simulink model "Threephase_diode_bridge_rectifier"  (R2022b)
settings: Solver=VariableStepAuto  StartTime=0.0  StopTime=10.0  RelTol=1e-3
libraries: spsDiodeLib x6, spsACVoltageSourceLib x3, spsMultimeterLib x3, spsSeriesRLCBranchLib x1, sps_lib x1
settings Model: Creator=vs632  LastModifiedBy=vs632

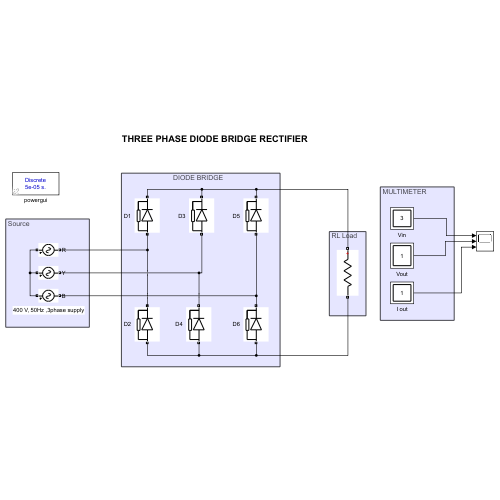
[thumbnail: Simulink's stored preview of the top-level diagram]
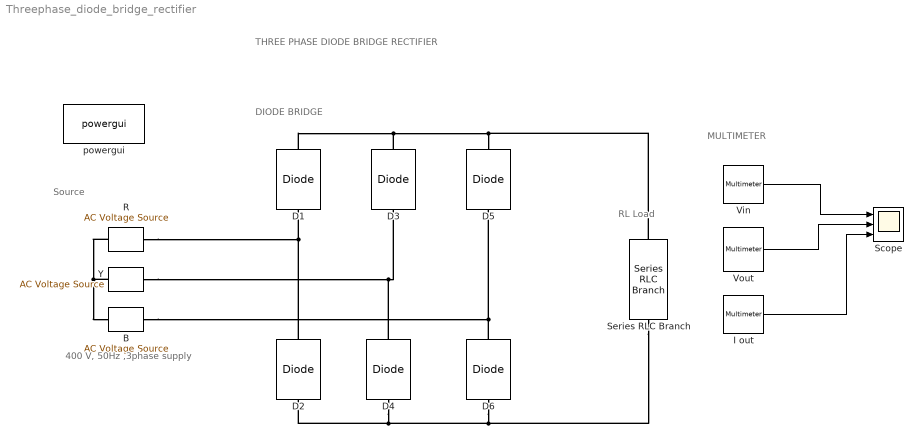
== system Threephase_diode_bridge_rectifier ==
  note: THREE PHASE DIODE BRIDGE RECTIFIER
  note: MULTIMETER
  note: Source
  note: RL Load
  note: DIODE BRIDGE
  note: 400 V, 50Hz ,3phase supply
  B : spsACVoltageSourceLib/AC Voltage Source  Amplitude=400  Phase=240  Frequency=60  SampleTime=0  Measurements=Voltage  BusType=swing  Pref=10e3  Qref=0  Qmin=-inf  Qmax=+inf
  D{1..6} (6 alike) : spsDiodeLib/Diode  Ron=0.001  Lon=0  Vf=0.8  IC=0  UseSnubber=0  Rs=500  Cs=250e-9  Measurements=off
  I out : spsMultimeterLib/Multimeter  L=5  sel=5  yselected={}  Gain=1  OutputType=Complex  PlotAtSimulationStop=off  PhasorSimulation=off
  R : spsACVoltageSourceLib/AC Voltage Source  Amplitude=400  Phase=0  Frequency=60  SampleTime=0  Measurements=Voltage  BusType=swing  Pref=10e3  Qref=0  Qmin=-inf  Qmax=+inf
  Scope : Scope  NumInputPorts=3
  Series RLC Branch : spsSeriesRLCBranchLib/Series RLC Branch  LConnTagsString=__new0  RConnTagsString=__new0  BranchType=R  Resistance=100  Inductance=15e-3  SetiL0=off  InitialCurrent=0  Capacitance=1e-6  Setx0=off  InitialVoltage=0  Measurements=Branch voltage and current
  Vin : spsMultimeterLib/Multimeter  L=5  sel=[2 3 4]  yselected={}  Gain=[1 1 1]  OutputType=Complex  PlotAtSimulationStop=off  PhasorSimulation=off
  Vout : spsMultimeterLib/Multimeter  L=5  sel=1  yselected={}  Gain=1  OutputType=Complex  PlotAtSimulationStop=off  PhasorSimulation=off
  Y : spsACVoltageSourceLib/AC Voltage Source  Amplitude=400  Phase=120  Frequency=60  SampleTime=0  Measurements=Voltage  BusType=swing  Pref=10e3  Qref=0  Qmin=-inf  Qmax=+inf
  powergui : sps_lib/powergui  Priority=1  SimulationMode=Discrete  SampleTime=50e-6  frequency=60  Iterations=50  frequencyindice=60  Pbase=100e6  ErrMax=1e-4  UnitsV=kV  UnitsW=MW  buscounter=0  FunctionMessages=off  echomessages=off  EnableUseOfTLC=off  CurrentSourceSwitches=off  DisableSnubberDevices=off  DisableRonSwitches=off  DisableVfSwitches=off  DisplayEquations=off  AutomaticDiscreteSolvers=off  SolverType=Tustin/Backward Euler (TBE)  Interpol=off  ExternalGateDelay=off  methode=off  Ts=100  x0status=blocks  SPID=on  SwTol=0  HookPort=off  NonlinearTolerance=1e-4  nMaxIteration=100  ContinueOnMaxIteration=off  RestoreLinks=warning  ResistiveCurrentMeasurement=off  Frange=[0:2:500]  Ylog=off  Xlog=on  ShowGrid=off  save=off  variable=ZData  structure=0  ZoomFFT=off  StartTime=0.0  cycles=1  DisplayStyle=1  fundamental=60  FreqAxis=off  MaxFrequency=1000  frequencyindicesteady=1  RmsSteady=1  display=off
  wires:
  Vout/1 -> Scope/2
  Vin/1 -> Scope/1
  I out/1 -> Scope/3
  connections:
  D2/RConn1 -- R/LConn1 -- D1/LConn1
  D4/RConn1 -- Y/LConn1 -- D3/LConn1
  D6/RConn1 -- B/LConn1 -- D5/LConn1
  D1/RConn1 -- D3/RConn1 -- Series RLC Branch/LConn1 -- D5/RConn1
  D6/LConn1 -- Series RLC Branch/RConn1 -- D2/LConn1 -- D4/LConn1
  R/RConn1 -- B/RConn1 -- Y/RConn1
